simulink model "Subsystem1"  (R2020b)
settings: Solver=VariableStepAuto  StartTime=0.0  StopTime=10.0  RelTol=1e-3
settings Model: DataDictionary=W2P4_dd.sldd  Creator=saadh  LastModifiedBy=saadh
settings DataIOCC: SaveOutput=off  SaveTime=off
settings DebuggingCC: AlgebraicLoopMsg=none

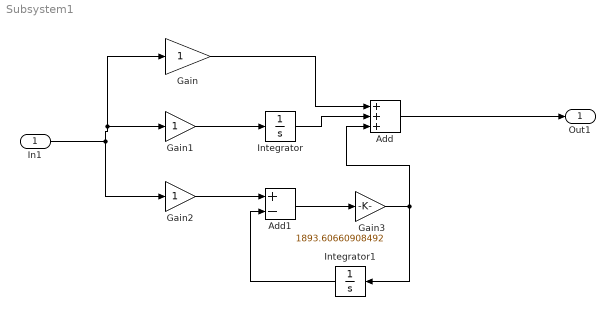
== system Subsystem1 ==
  In1 : Inport  OutDataTypeStr=double  PortDimensions=1  SampleTime=0
  Add : Sum  Inputs=+++
  Add1 : Sum  Inputs=+-
  Gain : Gain  mask{Kp=18.8618161296239}
  Gain1 : Gain  mask{Ki=554.412400621923}
  Gain2 : Gain  mask{Kd=0.154124143680084}
  Gain3 : Gain  Gain=1893.60660908492
  Integrator : Integrator
  Integrator1 : Integrator
  Out1 : Outport  OutDataTypeStr=double  PortDimensions=1  SampleTime=0
  wires:
  In1/1 -> Gain2/1, Gain1/1, Gain/1
  Gain/1 -> Add/1
  Gain1/1 -> Integrator/1
  Add/1 -> Out1/1
  Integrator/1 -> Add/2
  Gain2/1 -> Add1/1
  Add1/1 -> Gain3/1
  Gain3/1 -> Integrator1/1, Add/3
  Integrator1/1 -> Add1/2
